simulink model "mechatronics_ass1_q2"  (R2019a)
settings: Solver=VariableStepAuto  StartTime=0.0  StopTime=100  RelTol=1e-3
values from neighbouring files (symbols this model uses):
  K = 4    [adaptive_control_workspace.m]
  k1 = 10    [adaptive_control_workspace.m]
  k2 = 10    [adaptive_control_workspace.m]
  lamda_0 = 7    [adaptive_control_workspace.m]
  lamda_1 = 4    [adaptive_control_workspace.m]
  lamda_2 = 8.4    [adaptive_control_workspace.m]
  m = 10    [adaptive_control_workspace.m]
settings Model: Creator=ronil  LastModifiedBy=ronil

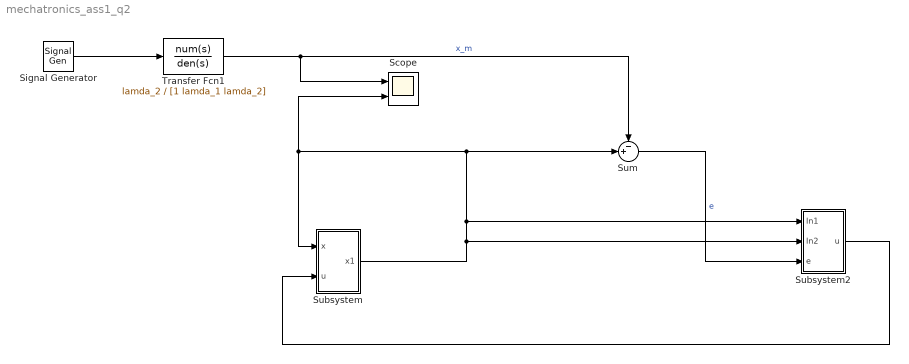
== system mechatronics_ass1_q2 ==
  Scope : Scope  NumInputPorts=2
  Signal Generator : SignalGenerator  Frequency=0.5  Units=rad/sec
  Subsystem : Subsystem
  Subsystem2 : Subsystem
  Sum : Sum  Inputs=-+|
  Transfer Fcn1 : TransferFcn  Numerator=lamda_2  Denominator=[1 lamda_1 lamda_2]
  wires:
  Transfer Fcn1/1 -> Sum/1, Scope/1  "x_m"
  Subsystem/1(x1) -> Subsystem2/2(In2), Subsystem2/1(In1), Sum/2, Scope/2, Subsystem/1(x)
  Signal Generator/1 -> Transfer Fcn1/1
  Sum/1 -> Subsystem2/3(e)  "e"
  Subsystem2/1(u) -> Subsystem/2(u)

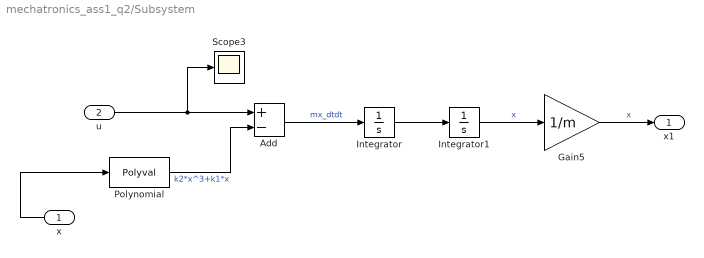
== system mechatronics_ass1_q2/Subsystem ==
  x : Inport
  u : Inport  Port=2
  Add : Sum  Inputs=+-
  Gain5 : Gain  Gain=1/m
  Integrator : Integrator
  Integrator1 : Integrator
  Polynomial : Polyval  Coefs=[k2 0 k1 0]
  Scope3 : Scope
  x1 : Outport
  wires:
  Integrator/1 -> Integrator1/1
  Integrator1/1 -> Gain5/1  "x"
  Polynomial/1 -> Add/2  "k2*x^3+k1*x"
  x/1 -> Polynomial/1
  u/1 -> Add/1, Scope3/1
  Add/1 -> Integrator/1  "mx_dtdt"
  Gain5/1 -> x1/1  "x"

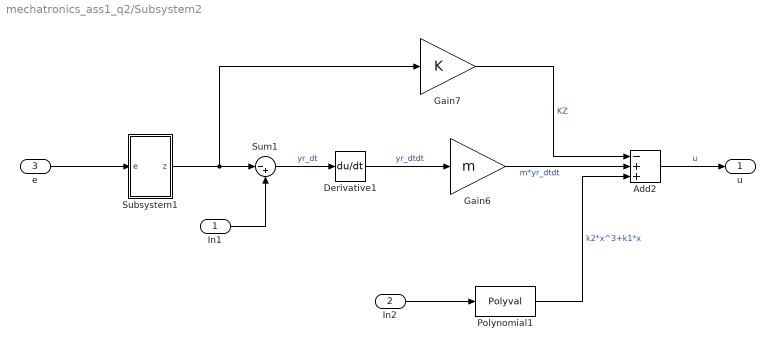
== system mechatronics_ass1_q2/Subsystem2 ==
  In1 : Inport
  In2 : Inport  Port=2
  e : Inport  Port=3
  Add2 : Sum  Inputs=-++
  Derivative1 : Derivative
  Gain6 : Gain  Gain=m
  Gain7 : Gain  Gain=K
  Polynomial1 : Polyval  Coefs=[k2 0 k1 0]
  Subsystem1 : Subsystem
  Sum1 : Sum  Inputs=|-+
  u : Outport
  wires:
  Gain6/1 -> Add2/2  "m*yr_dtdt"
  Sum1/1 -> Derivative1/1  "yr_dt"
  Subsystem1/1(z) -> Gain7/1, Sum1/1
  Derivative1/1 -> Gain6/1  "yr_dtdt"
  Gain7/1 -> Add2/1  "KZ"
  Polynomial1/1 -> Add2/3  "k2*x^3+k1*x"
  Add2/1 -> u/1  "u"
  In2/1 -> Polynomial1/1
  e/1 -> Subsystem1/1(e)
  In1/1 -> Sum1/2

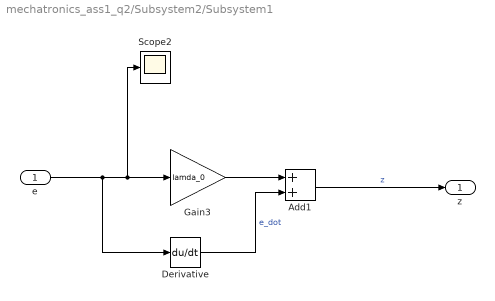
== system mechatronics_ass1_q2/Subsystem2/Subsystem1 ==
  e : Inport
  Add1 : Sum
  Derivative : Derivative
  Gain3 : Gain  Gain=lamda_0
  Scope2 : Scope
  z : Outport
  wires:
  e/1 -> Derivative/1, Scope2/1, Gain3/1
  Gain3/1 -> Add1/1
  Derivative/1 -> Add1/2  "e_dot"
  Add1/1 -> z/1  "z"
